simulink model "TestYaw"  (R2013b)
settings: Solver=ode45  StartTime=0.0  StopTime=200  RelTol=1e-8  AbsTol=1e-9
values from neighbouring files (symbols this model uses):
  G = tf(1/T , [1 0 1 0])    [ApPitch.m]    (also in ApYaw.m = 0.1)
  Iax = 1    [ApPitch.m]    (also in ApYaw.m)
  Ka = 1000    [ApPitch.m]    (also in ApYaw.m = 0.832562442183)
  Kq = -(p1 + p2 + p3)    (= -7)    [ApYaw.m]    (also in AutoPilot.m)
  Kss = 1    [ApYaw.m]
  Ksyn = -(p3*p1 + p3*p2 + p1*p2)  - Kq    (= -8)    [ApYaw.m]    (also in AutoPilot.m)
settings Model: Creator=Walker  LastModifiedBy=Walker

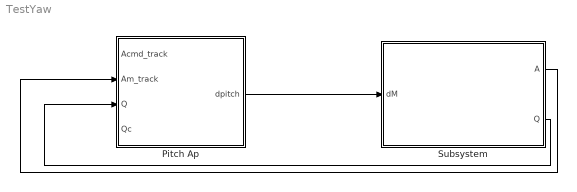
== system TestYaw ==
  Pitch Ap : Subsystem
  Subsystem : Subsystem
  wires:
  Pitch Ap/1(dpitch) -> Subsystem/1(dM)
  Subsystem/1(A) -> Pitch Ap/2(Am_track)
  Subsystem/2(Q) -> Pitch Ap/3(Q)

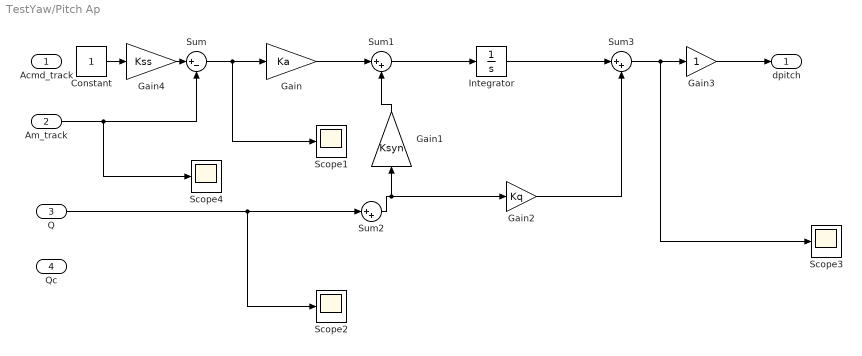
== system TestYaw/Pitch Ap ==
  Acmd_track : Inport
  Am_track : Inport  Port=2
  Q : Inport  Port=3
  Qc : Inport  Port=4
  Constant : Constant
  Gain : Gain  Gain=Ka
  Gain1 : Gain  Gain=Ksyn
  Gain2 : Gain  Gain=Kq
  Gain3 : Gain
  Gain4 : Gain  Gain=Kss
  Integrator : Integrator
  Scope{1..4} (4 alike) : Scope
      Scope1 settings: TimeRange=50  YMin=0.9  YMax=1.1  SaveName=ScopeData15
      Scope2 settings: TimeRange=50  YMin=-275  YMax=-75  SaveName=ScopeData21
      Scope3 settings: TimeRange=50  YMin=140  YMax=182.5  SaveName=ScopeData12
      Scope4 settings: TimeRange=50  YMin=0  YMax=35  SaveName=ScopeData25
  Sum : Sum  Inputs=|+-
  Sum1 : Sum  Inputs=|++
  Sum2 : Sum  Inputs=|++
  Sum3 : Sum  Inputs=|++
  dpitch : Outport
  wires:
  Am_track/1 -> Scope4/1, Sum/2
  Q/1 -> Scope2/1, Sum2/1
  Sum2/1 -> Gain2/1, Gain1/1
  Gain1/1 -> Sum1/2
  Sum1/1 -> Integrator/1
  Gain/1 -> Sum1/1
  Sum/1 -> Scope1/1, Gain/1
  Integrator/1 -> Sum3/1
  Gain2/1 -> Sum3/2
  Sum3/1 -> Gain3/1, Scope3/1
  Gain3/1 -> dpitch/1
  Constant/1 -> Gain4/1
  Gain4/1 -> Sum/1

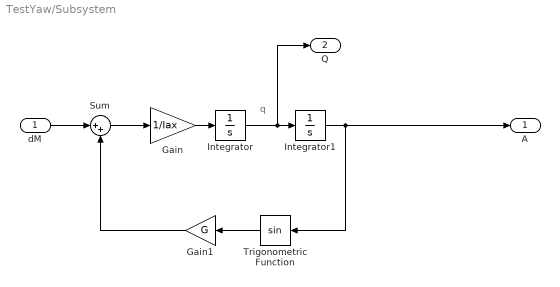
== system TestYaw/Subsystem ==
  note: q
  dM : Inport
  Gain : Gain  Gain=1/Iax
  Gain1 : Gain  Gain=G
  Integrator : Integrator
  Integrator1 : Integrator
  Sum : Sum  Inputs=|++
  Trigonometric Function : Trigonometry
  A : Outport
  Q : Outport  Port=2
  wires:
  dM/1 -> Sum/1
  Sum/1 -> Gain/1
  Gain/1 -> Integrator/1
  Integrator/1 -> Q/1, Integrator1/1
  Trigonometric Function/1 -> Gain1/1
  Gain1/1 -> Sum/2
  Integrator1/1 -> A/1, Trigonometric Function/1
